simulink model "testerWSimFeedbackLAG"  (R2018a)
settings: Solver=FixedStepAuto  StartTime=0.0  StopTime=200  FixedStep=.1  MaxStep=0.1  RelTol=1e-8
InitFcn:
  | %RLDesignJoystick
  | 
  | %divided K2 by 100, too small
  | %multiplied K2 by 10, needed damping
  | %multiplied b2 by 10, wrong direction
  | %divided original b2 by 2, getting better
  | %doubled K2
  | %double K2 again
  | %changed b2 to 0.2
  | b2=0.2667;
  | a2=35;
  | K2=1619.4;
  | %K2=809.9;
  | 
  | load('joystick_ref_002.mat')
  | 
  | % T = 20;
  | a = 10;
  | b = 0.4;
  | kp=1;
  | 
  | TD = 0.1;
  | 
  | sigma=0.5;
  | 
  | % SM Gains
  | k0 = 20;
  | k1 = 0.05;
  | 
  | % DAS
  | DT=2;
  | % gamma1sq=0.05;
  | % gamma2sq=0.3;
  | %sim parameters
  | %gamma1sq=0.025;
  | %gamma2sq=.015
  | 
  | %gamma1sq=0.025;
  | %gamma2sq=.07;
  | 
  | gamma1sq=-0.01;
  | gamma2sq=.005
  | 
  | y_ref=0;
  | 
  | 
  | %initSub = rossubscriber('/ship/state');
  | %initMsg = receive(initSub,10)
  | 
  | %Yd_init=initMsg.Pose.X
undefined symbols (not defined in the file or in its folder): DiscIntNeverNeededParam
libraries: simulink x8, robotlib x3, vrlib x1, peGeneralControl x1
settings Model: SimulationMode=accelerator  EnablePacing=on  Creator=KvonEllenrieder  LastModifiedBy=transmogrifier
settings SolverCC: ZeroCrossAlgorithm=Adaptive
settings OptimizationCC: EfficientMapNaN2IntZero=off
settings DebuggingCC: IgnoredZcDiagnostic=none
settings HardwareCC: TargetBitPerLong=64  TargetBitPerPointer=64  TargetBitPerSizeT=64  TargetBitPerPtrDiffT=64  TargetLongLongMode=on  TargetIntDivRoundTo=Zero  TargetEndianess=LittleEndian  TargetWordSize=64  TargetHWDeviceType=MATLAB Host  ProdEqTarget=off
settings CodeAppCC: MaxIdLength=128
settings GRTTargetCC: TargetLangStandard=C89/C90 (ANSI)  CombineOutputUpdateFcns=off  GRTInterface=on

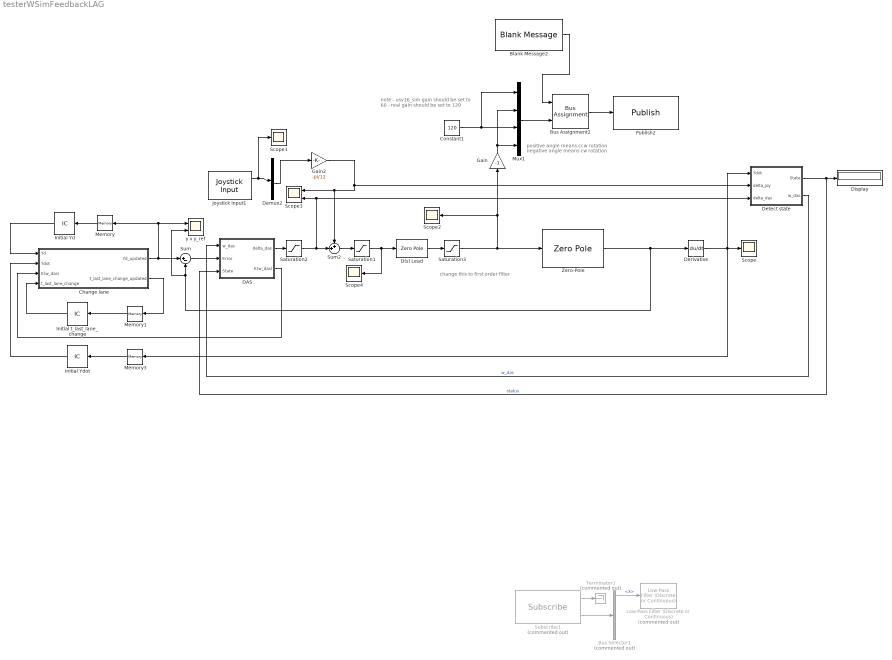
== system testerWSimFeedbackLAG ==
  note: change this to first order filter
  note: positive angle means ccw rotation
      | negative angle means cw rotation
  note: note
      |  - usv16_sim gain should be set to 60
      |  - real gain should be set to 120
  Blank Message2 : robotlib/Blank Message  SourceLibraryInfo=This block requires Robotics System Toolbox  messageType=usv16_msgs/Usv16ActuatorInputs  SampleTime=.1
      settings: SourceProductBaseCode=RO
  Bus Assignment2 : BusAssignment  AssignedSignals=ActuatorInputs
  Bus Selector1 : BusSelector  Commented=on  OutputSignals=Pose.X,Pose.Y,Vel.Linear.X,Vel.Linear.Y
  Change lane : Subsystem
  Constant1 : Constant  Value=120
  D(s) Lead : ZeroPole  Zeros=[-.26]  Poles=[-3]  Gain=[60]
  DAS : Subsystem
  Demux2 : Demux  Outputs=6
  Derivative : Derivative
  Detect state : Subsystem
  Display : Display
  Gain : Gain  Gain=-1
  Gain2 : Gain  Gain=-pi/12
  Initial Yd : InitialCondition  Value=0
  Initial Ydot : InitialCondition  Value=0
  Initial t_last_lane_change : InitialCondition  Value=0
  Joystick Input1 : vrlib/Joystick Input  joyid=1  adjustports=on  forcefeed=off
      settings: SourceProductBaseCode=VR
  Low-Pass Filter (Discrete or Continuous) : peGeneralControl/Low-Pass Filter (Discrete or Continuous)  Commented=on  K=1  T=0.808  B=inf  A=-inf  Ts=0.1
  Memory : Memory
  Memory1 : Memory
  Memory3 : Memory
  Mux1 : Mux
  Publish2 : robotlib/Publish  SourceLibraryInfo=This block requires Robotics System Toolbox  topicSource=Select from ROS network  topic=/ship/actuation  messageType=usv16_msgs/Usv16ActuatorInputs  messageQueueLength=1
      settings: SourceProductBaseCode=RO
  Saturation1 : Saturate  UpperLimit=pi/12  LowerLimit=-pi/12
  Saturation2 : Saturate  UpperLimit=pi/12  LowerLimit=-pi/12
  Saturation3 : Saturate  UpperLimit=pi/12  LowerLimit=-pi/12
  Scope{,1..2,4} (4 alike) : Scope
  Scope3 : Scope  NumInputPorts=2
  Subscribe1 : robotlib/Subscribe  Commented=on  SourceLibraryInfo=This block requires Robotics System Toolbox  topicSource=Select from ROS network  topic=/ship/state  messageType=usv16_msgs/Usv16State  sampleTime=.1  messageQueueLength=1
      settings: SourceProductBaseCode=RO
  Sum : Sum  Inputs=|+-
  Sum2 : Sum  Inputs=++|
  Terminator1 : Terminator  Commented=on
  Zero-Pole : ZeroPole  Zeros=[]  Poles=[0 0 -5/4]  Gain=3
  y v y_ref : Scope  NumInputPorts=2
  wires:
  Joystick Input1/1 -> Scope1/1, Demux2/1
  Constant1/1 -> Mux1/1, Mux1/3
  DAS/1(delta_das) -> Saturation2/1
  Demux2/4 -> Gain2/1
  Initial Yd/1 -> Change lane/1(Yd)
  Memory3/1 -> Initial Ydot/1
  DAS/2(K(w_das)) -> Change lane/3(K(w_das))
  Change lane/1(Yd_updated) -> Memory/1, y v y_ref/1, Sum/1
  Change lane/2(t_last_lane_change_updated) -> Memory1/1
  Initial Ydot/1 -> Change lane/2(Ydot)
  Detect state/2(w_das) -> DAS/1(w_das)  "w_das"
  Blank Message2/1 -> Bus Assignment2/1
  Memory1/1 -> Initial t_last_lane_change/1
  Sum2/1 -> Saturation1/1
  Detect state/1(State) -> Display/1, DAS/3(State)  "status"
  Mux1/1 -> Bus Assignment2/2
  Sum/1 -> DAS/2(Error)
  D(s) Lead/1 -> Saturation3/1
  Initial t_last_lane_change/1 -> Change lane/4(t_last_lane_change)
  Memory/1 -> Initial Yd/1
  Bus Assignment2/1 -> Publish2/1
  Gain/1 -> Mux1/4, Mux1/2
  Derivative/1 -> Detect state/1(Ydot), Scope/1, Memory3/1
  Zero-Pole/1 -> Derivative/1, y v y_ref/2, Sum/2
  Gain2/1 -> Sum2/1, Scope3/1, Detect state/2(delta_joy)
  Saturation2/1 -> Sum2/2, Detect state/3(delta_das), Scope3/2
  Subscribe1/2 -> Bus Selector1/1
  Subscribe1/1 -> Terminator1/1
  Bus Selector1/1 -> Low-Pass Filter (Discrete or Continuous)/1  "<X>"
  Saturation3/1 -> Zero-Pole/1, Scope2/1, Gain/1
  Saturation1/1 -> D(s) Lead/1, Scope4/1

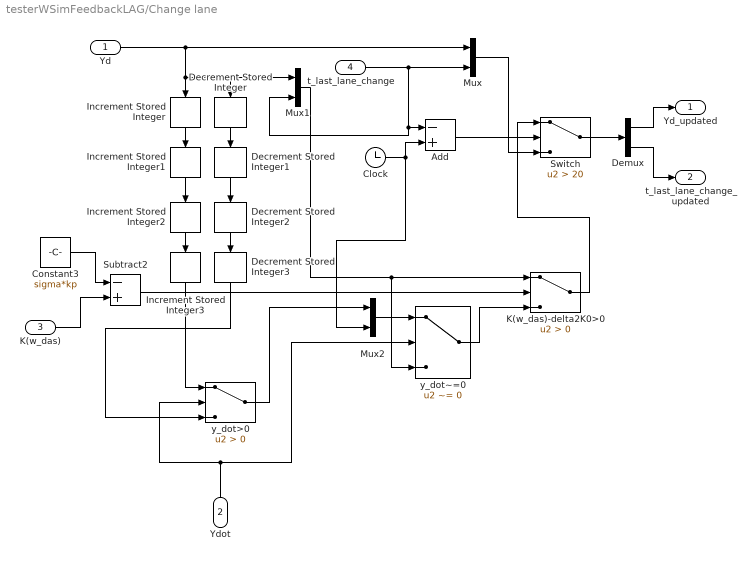
== system testerWSimFeedbackLAG/Change lane ==
  Yd : Inport
  Ydot : Inport  Port=2
  K(w_das) : Inport  Port=3
  t_last_lane_change : Inport  Port=4
  Add : Sum  Inputs=-+
  Clock : Clock
  Constant3 : Constant  Value=sigma*kp
  Decrement Stored Integer{,1..3} (4 alike) : simulink/Additional Math & Discrete/Additional Math: Increment - Decrement/Decrement Stored Integer
      settings: SourceProductName=Simulink  SourceProductBaseCode=SL
  Demux : Demux  Outputs=2
  Increment Stored Integer{,1..3} (4 alike) : simulink/Additional Math & Discrete/Additional Math: Increment - Decrement/Increment Stored Integer
      settings: SourceProductName=Simulink
  K(w_das)-delta2K0>0 : Switch  Criteria=u2 > Threshold  ZeroCross=off
  Mux : Mux  Inputs=2
  Mux1 : Mux  Inputs=2
  Mux2 : Mux  Inputs=2
  Subtract2 : Sum  Inputs=-+
  Switch : Switch  Criteria=u2 > Threshold  Threshold=20
  y_dot>0 : Switch  Criteria=u2 > Threshold
  y_dot~=0 : Switch  Criteria=u2 ~= 0
  Yd_updated : Outport
  t_last_lane_change_updated : Outport  Port=2
  wires:
  Increment Stored Integer/1 -> Increment Stored Integer1/1
  y_dot>0/1 -> Mux2/1
  K(w_das)/1 -> Subtract2/2
  Yd/1 -> Mux/1, Mux1/1, Decrement Stored Integer/1, Increment Stored Integer/1
  y_dot~=0/1 -> K(w_das)-delta2K0>0/3
  Constant3/1 -> Subtract2/1
  Ydot/1 -> y_dot~=0/2, y_dot>0/2
  Decrement Stored Integer/1 -> Decrement Stored Integer1/1
  Clock/1 -> Mux2/2, Add/2
  t_last_lane_change/1 -> Mux1/2, Add/1, Mux/2
  Add/1 -> Switch/2
  K(w_das)-delta2K0>0/1 -> Switch/1
  Mux/1 -> Switch/3
  Switch/1 -> Demux/1
  Demux/1 -> Yd_updated/1
  Demux/2 -> t_last_lane_change_updated/1
  Mux1/1 -> K(w_das)-delta2K0>0/1, y_dot~=0/3
  Mux2/1 -> y_dot~=0/1
  Subtract2/1 -> K(w_das)-delta2K0>0/2
  Increment Stored Integer1/1 -> Increment Stored Integer2/1
  Increment Stored Integer2/1 -> Increment Stored Integer3/1
  Increment Stored Integer3/1 -> y_dot>0/1
  Decrement Stored Integer1/1 -> Decrement Stored Integer2/1
  Decrement Stored Integer2/1 -> Decrement Stored Integer3/1
  Decrement Stored Integer3/1 -> y_dot>0/3

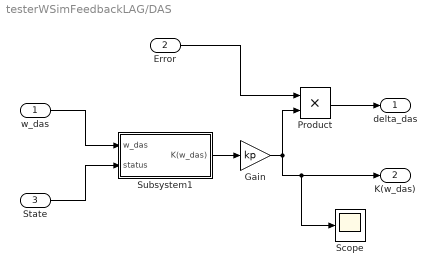
== system testerWSimFeedbackLAG/DAS ==
  w_das : Inport
  Error : Inport  Port=2
  State : Inport  Port=3
  Gain : Gain  Gain=kp
  Product : Product
  Scope : Scope
  Subsystem1 : Subsystem
  delta_das : Outport
  K(w_das) : Outport  Port=2
  wires:
  Product/1 -> delta_das/1
  Error/1 -> Product/1
  State/1 -> Subsystem1/2(status)
  Subsystem1/1(K(w_das)) -> Gain/1
  Gain/1 -> Product/2, Scope/1, K(w_das)/1
  w_das/1 -> Subsystem1/1(w_das)

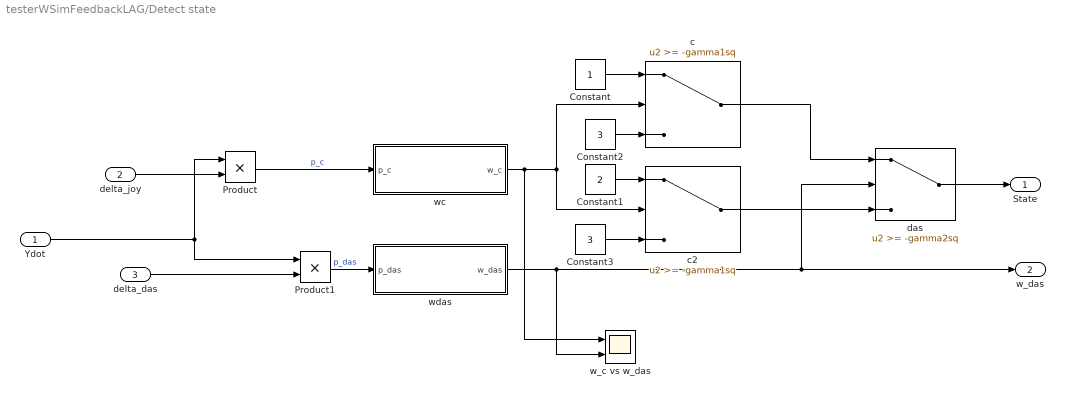
== system testerWSimFeedbackLAG/Detect state ==
  Ydot : Inport
  delta_joy : Inport  Port=2
  delta_das : Inport  Port=3
  Constant : Constant
  Constant1 : Constant  Value=2
  Constant2 : Constant  Value=3
  Constant3 : Constant  Value=3
  Product : Product
  Product1 : Product
  c : Switch  Threshold=-gamma1sq
  c2 : Switch  Threshold=-gamma1sq
  das : Switch  Threshold=-gamma2sq
  w_c vs w_das : Scope  NumInputPorts=2
  wc : Subsystem
  wdas : Subsystem
  State : Outport
  w_das : Outport  Port=2
  wires:
  Ydot/1 -> Product/1, Product1/1
  delta_joy/1 -> Product/2
  delta_das/1 -> Product1/2
  Product/1 -> wc/1(p_c)  "p_c"
  Product1/1 -> wdas/1(p_das)  "p_das"
  wdas/1(w_das) -> w_c vs w_das/2, w_das/1, das/2
  wc/1(w_c) -> w_c vs w_das/1, c2/2, c/2
  Constant/1 -> c/1
  c/1 -> das/1
  Constant1/1 -> c2/1
  c2/1 -> das/3
  Constant3/1 -> c2/3
  Constant2/1 -> c/3
  das/1 -> State/1

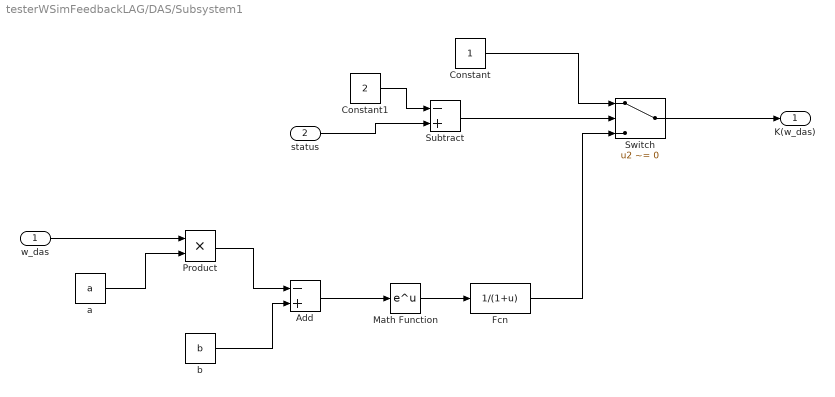
== system testerWSimFeedbackLAG/DAS/Subsystem1 ==
  w_das : Inport
  status : Inport  Port=2
  Add : Sum  Inputs=-+
  Constant : Constant
  Constant1 : Constant  Value=2
  Fcn : Fcn  Expr=1/(1+u)
  Math Function : Math  SaturateOnIntegerOverflow=on
  Product : Product
  Subtract : Sum  Inputs=-+
  Switch : Switch  Criteria=u2 ~= 0
  a : Constant  Value=a
  b : Constant  Value=b
  K(w_das) : Outport
  wires:
  w_das/1 -> Product/1
  a/1 -> Product/2
  Product/1 -> Add/1
  b/1 -> Add/2
  Add/1 -> Math Function/1
  Math Function/1 -> Fcn/1
  Fcn/1 -> Switch/3
  Constant/1 -> Switch/1
  Switch/1 -> K(w_das)/1
  Constant1/1 -> Subtract/1
  status/1 -> Subtract/2
  Subtract/1 -> Switch/2

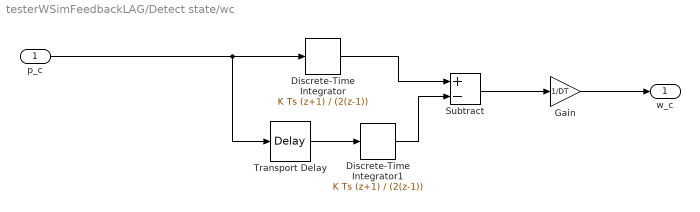
== system testerWSimFeedbackLAG/Detect state/wc ==
  p_c : Inport
  Discrete-Time Integrator : DiscreteIntegrator  IntegratorMethod=Integration: Trapezoidal  SampleTime=.1  ICPrevOutput=DiscIntNeverNeededParam  ICPrevScaledInput=DiscIntNeverNeededParam
  Discrete-Time Integrator1 : DiscreteIntegrator  IntegratorMethod=Integration: Trapezoidal  SampleTime=.1  ICPrevOutput=DiscIntNeverNeededParam  ICPrevScaledInput=DiscIntNeverNeededParam
  Gain : Gain  Gain=1/DT
  Subtract : Sum  Inputs=+-
  Transport Delay : TransportDelay  DelayTime=DT  TransDelayFeedthrough=on
  w_c : Outport
  wires:
  p_c/1 -> Discrete-Time Integrator/1, Transport Delay/1
  Discrete-Time Integrator/1 -> Subtract/1
  Transport Delay/1 -> Discrete-Time Integrator1/1
  Gain/1 -> w_c/1
  Subtract/1 -> Gain/1
  Discrete-Time Integrator1/1 -> Subtract/2

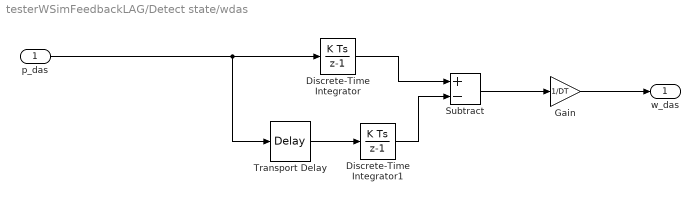
== system testerWSimFeedbackLAG/Detect state/wdas ==
  p_das : Inport
  Discrete-Time Integrator : DiscreteIntegrator  SampleTime=.1  ICPrevOutput=DiscIntNeverNeededParam  ICPrevScaledInput=DiscIntNeverNeededParam
  Discrete-Time Integrator1 : DiscreteIntegrator  SampleTime=.1  ICPrevOutput=DiscIntNeverNeededParam  ICPrevScaledInput=DiscIntNeverNeededParam
  Gain : Gain  Gain=1/DT
  Subtract : Sum  Inputs=+-
  Transport Delay : TransportDelay  DelayTime=DT  FixedBuffer=on
  w_das : Outport
  wires:
  Subtract/1 -> Gain/1
  Gain/1 -> w_das/1
  Transport Delay/1 -> Discrete-Time Integrator1/1
  Discrete-Time Integrator1/1 -> Subtract/2
  Discrete-Time Integrator/1 -> Subtract/1
  p_das/1 -> Discrete-Time Integrator/1, Transport Delay/1
